simulink model "sliding_model"  (R2017a)
settings: Solver=VariableStepAuto  StartTime=0.0  StopTime=4  FixedStep=0.001  MaxStep=0.001  RelTol=1e-3
settings Model: Creator=tivay  LastModifiedBy=tivay

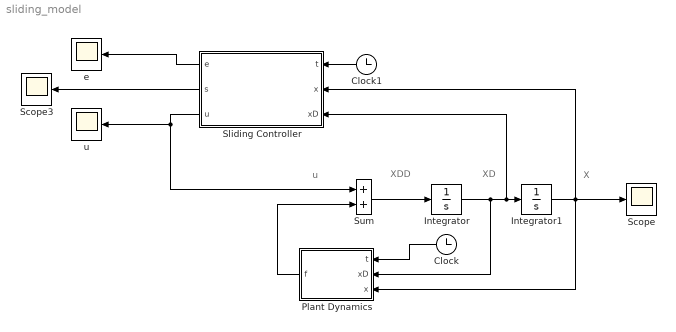
== system sliding_model ==
  note: u
  note: X
  note: XD
  note: XDD
  Clock : Clock
  Clock1 : Clock
  Integrator : Integrator  InitialCondition=1.5708
  Integrator1 : Integrator
  Plant Dynamics : MATLAB Function  TreatAsAtomicUnit=on
  Scope : Scope
  Scope3 : Scope
  Sliding Controller : MATLAB Function  TreatAsAtomicUnit=on
  Sum : Sum
  e : Scope
  u : Scope
  wires:
  Integrator/1 -> Sliding Controller/3(xD), Integrator1/1, Plant Dynamics/2(xD)
  Sum/1 -> Integrator/1
  Plant Dynamics/1(f) -> Sum/2
  Integrator1/1 -> Sliding Controller/2(x), Scope/1, Plant Dynamics/3(x)
  Clock/1 -> Plant Dynamics/1(t)
  Clock1/1 -> Sliding Controller/1(t)
  Sliding Controller/3(u) -> Sum/1, u/1
  Sliding Controller/1(e) -> e/1
  Sliding Controller/2(s) -> Scope3/1

== matlab function sliding_model/Sliding Controller ==
  data: e output; s output; t input; u output; x input; xD input
function [e,s,u] = fcn(t, x,xD)

    % parameters
    lambda = 20;
    eta = 0.1;

    % desired trajectory
    xd = sin(pi*t/2);
    xdD = (pi/2)*cos(pi*t/2);
    xdDD = -(pi/2)^2*sin(pi*t/2);
    
    % tracking error and derivatives
    e = x-xd;
    eD = xD-xdD;
    
    % nominal control
    uhat = 1.5*xD^2*cos(3*x)+xdDD-lambda*eD;
    
    % switching magnitude
    k = 0.5*xD^2*abs(cos(3*x)) + eta;
    
    % sliding surface
    s = eD + lambda*e;
    
    % control law
    u = uhat - k*sign(s);

end

== matlab function sliding_model/Plant Dynamics ==
  data: t input; xD input; x input; f output
function f = fcn(t,xD,x)

    % uncertainty
    a = 1 + abs(sin(t));
    
    % nonlinearity
    f = -a*xD^2*cos(3*x);
    
end
